simulink model "appint_minex_extmode"  (Simulink 9.2)
settings: Solver=FixedStepDiscrete  StartTime=0.0  StopTime=inf  FixedStep=1e-3  RelTol=1e-3
settings Model: Creator=moritz  LastModifiedBy=schappler  SimulationMode=external  ExtModeTrigDuration=10000  ExtModeArchiveMode=auto  ExtModeArchiveFileName=measurement_data  ExtModeArchiveDirName=./results
settings DataIOCC: LimitDataPoints=off  SaveFormat=Dataset  SignalLoggingSaveFormat=Dataset  SaveOutput=off  SignalLogging=off  SaveTime=off
settings OptimizationCC: BlockReduction=off  ConditionallyExecuteInputs=off  OptimizeBlockIOStorage=off  BufferReuse=off  GlobalBufferReuse=off  ExpressionFolding=off  LocalBlockOutputs=off  LifeSpan=auto  OptimizeDataStoreBuffers=off  BusAssignmentInplaceUpdate=off
settings DebuggingCC: UnderspecifiedInitializationDetection=Simplified  MergeDetectMultiDrivingBlocksExec=error  FcnCallInpInsideContextMsg=error  StateNameClashWarn=none  SFUnexpectedBacktrackingDiag=error  SFNoUnconditionalDefaultTransitionDiag=error  SFExecutionAtInitializationDiag=warning
settings HardwareCC: ProdBitPerPointer=64  ProdBitPerSizeT=64  ProdBitPerPtrDiffT=64  ProdLargestAtomicFloat=Float  ProdIntDivRoundTo=Zero  ProdEndianess=LittleEndian  ProdWordSize=64  ProdHWDeviceType=Intel->x86-64 (Windows64)
settings ModelReferenceCC: PropagateSignalLabelsOutOfModel=on
settings RTWCC: SystemTargetFile=etherlab.tlc  TemplateMakefile=etherlab_hrt.tmf  Description=EtherLab PREEMT_RT Real-Time Target
settings CodeAppCC: StateflowObjectComments=off
settings STFCustomTargetCC: TargetLangStandard=C99 (ISO)  SystemTargetFile=etherlab.tlc
settings GRTTargetCC: TargetLangStandard=C99 (ISO)  ParMdlRefBuildCompliant=off  CompOptLevelCompliant=off  ConcurrentExecutionCompliant=off  GeneratePreprocessorConditionals=Use local settings  MatFileLogging=off  CPPClassGenCompliant=off  UseToolchainInfoCompliant=off  ExtMode=on  ExtModeStaticAlloc=on  ExtModeStaticAllocSize=10000000  ExtModeMexArgs='10.144.130.83' 0 17725  RTWCAPISignals=on  RTWCAPIParams=on
settings CustomProperty: DataType=int32  Value=2
settings ConfigComp: CovMetricSettings=dwe  CovHtmlReporting=off  CovSaveCumulativeToWorkspaceVar=off  CovSaveSingleToWorkspaceVar=off  CovExternalEMLEnable=on

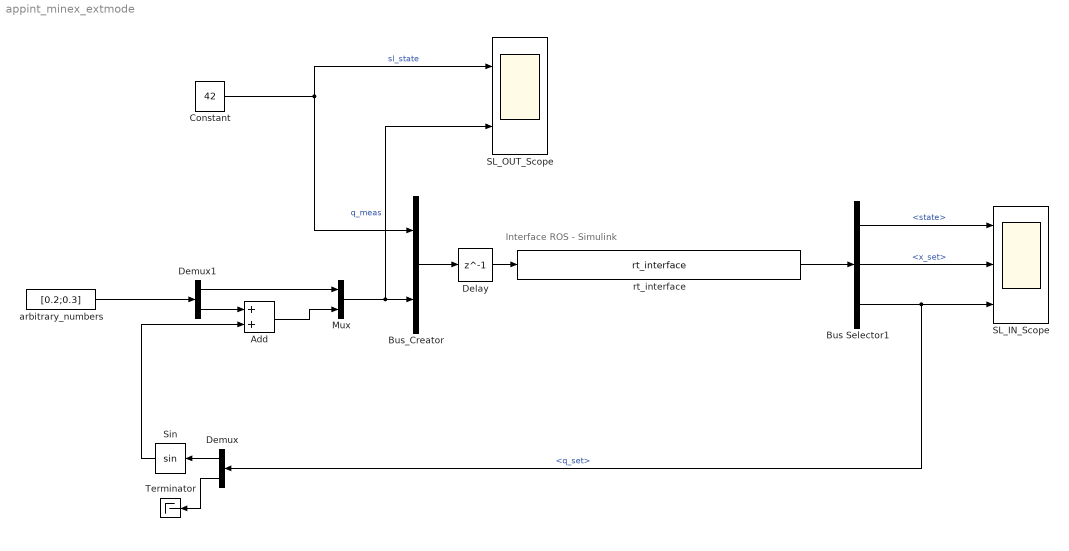
== system appint_minex_extmode ==
  note: Interface ROS - Simulink
  Add : Sum
  Bus Selector1 : BusSelector  OutputSignals=state,x_set,q_set
  Bus_Creator : BusCreator  Inputs=2
  Constant : Constant  Value=42  OutDataTypeStr=uint8
  Delay : Delay  DelayLength=1
  Demux : Demux  Outputs=2
  Demux1 : Demux  Outputs=2
  Mux : Mux  Inputs=2
  SL_IN_Scope : Scope  NumInputPorts=3
  SL_OUT_Scope : Scope  NumInputPorts=2
  Sin : Trigonometry
  Terminator : Terminator
  arbitrary_numbers : Constant  Value=[0.2;0.3]  OutDataTypeStr=double
  rt_interface : S-Function  FunctionName=rt_interface  SFunctionDeploymentMode=off  EnableBusSupport=off  mask(Legacy Function){SFunctionSpec=void SL_io_func(SL_OUT_type u1[1], SL_IN_type y1[1]), ShowSpec=on}
      mask prompts: ShowSpec "Display function specification"
      mask help:
      | This block allows you to call the legacy functions specified by the following Legacy Code Tool definition:
      | def.SFunctionName = 'rt_interface';
      | def.OutputFcnSpec = 'void SL_io_func(SL_OUT_type u1[1], SL_IN_type y1[1])';
      | def.StartFcnSpec = 'void SL_start_func()';
      | def.TerminateFcnSpec = 'void SL_terminate_func()';
      | def.HeaderFiles = {'SL_func.h'};
      | def.SourceFiles = {'../rt_interface/ros_rt_core/SL_func_dummy.cpp'};
      | def.TargetLibFiles = {'libros_sl_interface.so'};
      | def.IncPaths = {'../rt_interface/ros_rt_core'};
      mask Help: <p>This block was generated automatically by the Legacy Code Tool. For detailed help on this tool, call<a href="matlab:legacy_code('help')"> legacy_code('help')</a>.</p>
      mask Callback ShowSpec:
      | if strcmp(get_param(gcbh, 'ShowSpec'), 'on')
      |   set_param(gcbh, 'MaskDisplay', sprintf('fprintf(''%s'');', get_param(gcbh, 'SFunctionSpec')));
      | else
      |   set_param(gcbh, 'MaskDisplay', sprintf('fprintf(''%s'');', get_param(gcbh, 'FunctionName')));
      | end
      mask Display: fprintf('void SL_io_func(SL_OUT_type u1[1], SL_IN_type y1[1])');
  wires:
  Delay/1 -> rt_interface/1
  Bus_Creator/1 -> Delay/1
  rt_interface/1 -> Bus Selector1/1
  Constant/1 -> Bus_Creator/1, SL_OUT_Scope/1  "sl_state"
  arbitrary_numbers/1 -> Demux1/1
  Mux/1 -> SL_OUT_Scope/2, Bus_Creator/2  "q_meas"
  Bus Selector1/1 -> SL_IN_Scope/1  "<state>"
  Bus Selector1/2 -> SL_IN_Scope/2  "<x_set>"
  Bus Selector1/3 -> Demux/1, SL_IN_Scope/3  "<q_set>"
  Demux/1 -> Sin/1
  Sin/1 -> Add/2
  Demux/2 -> Terminator/1
  Demux1/2 -> Add/1
  Add/1 -> Mux/2
  Demux1/1 -> Mux/1
